simulink model "SplineGeneratorTest"  (R2016b)
settings: Solver=VariableStepAuto  StartTime=0.0  StopTime=10.0  RelTol=1e-3
settings Model: DataDictionary=DataDictionary.sldd  Creator=march  LastModifiedBy=Taeke

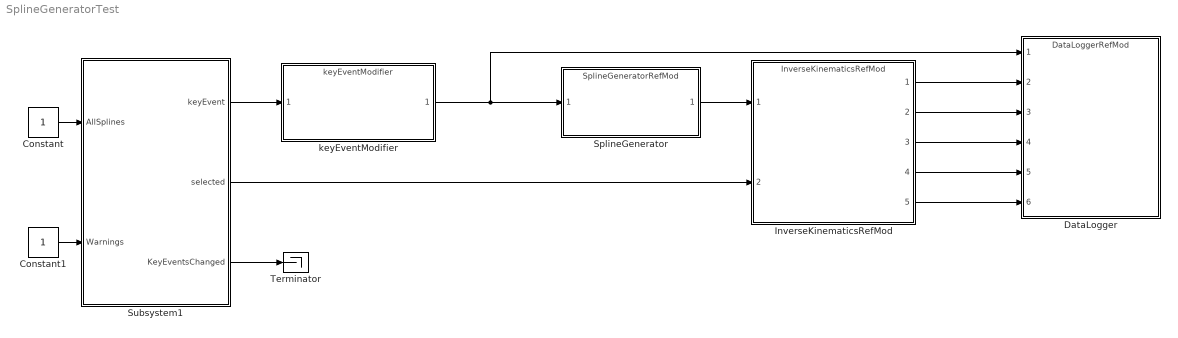
== system SplineGeneratorTest ==
  Constant : Constant
  Constant1 : Constant
  DataLogger : ModelReference  ModelNameDialog=DataLoggerRefMod.slx  SimulationMode=Normal  ModelReferenceVersion=1.16
  InverseKinematicsRefMod : ModelReference  ModelNameDialog=InverseKinematicsRefMod.slx  SimulationMode=Normal  ModelReferenceVersion=1.78
  SplineGenerator : ModelReference  ModelNameDialog=SplineGeneratorRefMod.slx  SimulationMode=Normal  ModelReferenceVersion=1.42
  Subsystem1 : Subsystem
  Terminator : Terminator
  keyEventModifier : ModelReference  ModelNameDialog=keyEventModifier.slx  SimulationMode=Normal  ModelReferenceVersion=1.7
  wires:
  Subsystem1/3(KeyEventsChanged) -> Terminator/1
  Constant/1 -> Subsystem1/1(AllSplines)
  Constant1/1 -> Subsystem1/2(Warnings)
  keyEventModifier/1 -> DataLogger/1, SplineGenerator/1
  SplineGenerator/1 -> InverseKinematicsRefMod/1
  Subsystem1/1(keyEvent) -> keyEventModifier/1
  Subsystem1/2(selected) -> InverseKinematicsRefMod/2
  InverseKinematicsRefMod/5 -> DataLogger/6
  InverseKinematicsRefMod/4 -> DataLogger/5
  InverseKinematicsRefMod/3 -> DataLogger/4
  InverseKinematicsRefMod/2 -> DataLogger/3
  InverseKinematicsRefMod/1 -> DataLogger/2

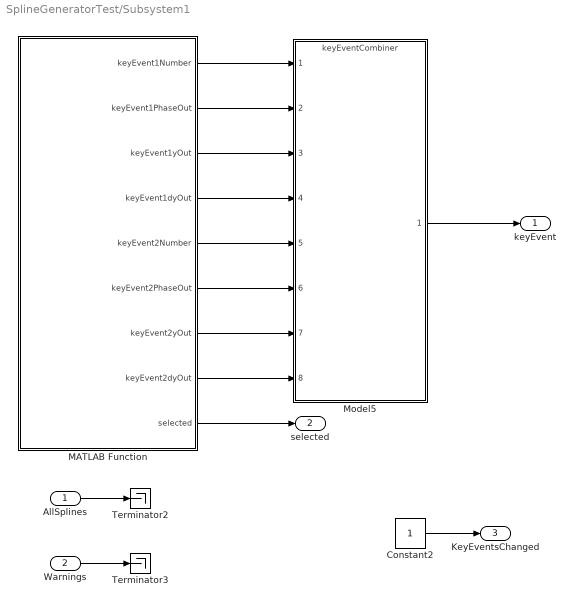
== system SplineGeneratorTest/Subsystem1 ==
  AllSplines : Inport
  Warnings : Inport  Port=2
  Constant2 : Constant
  MATLAB Function : MATLAB Function  TreatAsAtomicUnit=on
  Model5 : ModelReference  ModelNameDialog=keyEventCombiner.slx  SimulationMode=Normal  ModelReferenceVersion=1.6
  Terminator2 : Terminator
  Terminator3 : Terminator
  keyEvent : Outport
  selected : Outport  Port=2
  KeyEventsChanged : Outport  Port=3
  wires:
  Warnings/1 -> Terminator3/1
  MATLAB Function/8(keyEvent2dyOut) -> Model5/8
  AllSplines/1 -> Terminator2/1
  MATLAB Function/3(keyEvent1yOut) -> Model5/3
  Constant2/1 -> KeyEventsChanged/1
  MATLAB Function/4(keyEvent1dyOut) -> Model5/4
  MATLAB Function/2(keyEvent1PhaseOut) -> Model5/2
  MATLAB Function/6(keyEvent2PhaseOut) -> Model5/6
  MATLAB Function/1(keyEvent1Number) -> Model5/1
  MATLAB Function/7(keyEvent2yOut) -> Model5/7
  Model5/1 -> keyEvent/1
  MATLAB Function/5(keyEvent2Number) -> Model5/5
  MATLAB Function/9(selected) -> selected/1

== matlab function SplineGeneratorTest/Subsystem1/MATLAB Function ==
  data: keyEvent1Number output; keyEvent1PhaseOut output; keyEvent1yOut output; keyEvent1dyOut output; keyEvent2Number output; keyEvent2PhaseOut output; keyEvent2yOut output; keyEvent2dyOut output; selected output
function [keyEvent1Number, keyEvent1PhaseOut,keyEvent1yOut,keyEvent1dyOut, ...
    keyEvent2Number, keyEvent2PhaseOut,keyEvent2yOut,keyEvent2dyOut,...
    selected] = fcn()

selected1 = [0 ,1, 0, 0]; %[Hip, Knee, x, y];
selected2 = [0 ,0, 1, 0]; %[Hip, Knee, x, y];

selected = selected1 + selected2; %knee and x selected

keyEventHipPhase = [55, 85]; %hip angle: for test look_up_hip_y
keyEventHipAngle = [-7, 20]/180*pi; %hip angle: for test look_up_hip_y
keyEventHipdAngle = [0,0]; %hip angle: for test look_up_hip_y

keyEventKneePhase = [0, 18, 45, 78];   %knee angle: for test look_up_hip_y
keyEventKneeAngle = [0, 15, 2, 60]/180*pi;  %knee angle: for test look_up_hip_y 
keyEventKneedAngle = [0,0, 0 ,0]; %knee angle: for test look_up_hip_y

keyEventxPhase = [0, 18, 45, 62];
keyEventxPos = [0.15, 0.0, -0.1, -0.25]; %[m] x position: for test look_up_hip_y
keyEventxdPos = [0, -0.0035, -0.0035, 0]; % x position: for test look_up_hip_y

if selected1(1)
    keyEvent1Phase = keyEventHipPhase;
    keyEvent1y = keyEventHipAngle;
    keyEvent1dy = keyEventHipdAngle;
elseif selected1(2)
    keyEvent1Phase = keyEventKneePhase; 
    keyEvent1y = keyEventKneeAngle;
    keyEvent1dy = keyEventKneedAngle;
elseif selected1(3)  
    keyEvent1Phase = keyEventxPhase;
    keyEvent1y = keyEventxPos;
    keyEvent1dy = keyEventxdPos;
elseif selected1(4)    
    keyEvent1Phase = keyEventyPhase; 
    keyEvent1y = keyEventxPos;
    keyEvent1dy = keyEventxdAngle;
end

if selected2(1)
    keyEvent2Phase = keyEventHipPhase;
    keyEvent2y = keyEventHipAngle;
    keyEvent2dy = keyEventHipdAngle;
elseif selected2(2)
    keyEvent2Phase = keyEventKneePhase; 
    keyEvent2y = keyEventKneeAngle;
    keyEvent2dy = keyEventKneedAngle;
elseif selected2(3)  
    keyEvent2Phase = keyEventxPhase;
    keyEvent2y = keyEventxPos;
    keyEvent2dy = keyEventxdPos;
elseif selected2(4)    
    keyEvent2Phase = keyEventyPhase; 
    keyEvent2y = keyEventxPos;
    keyEvent2dy = keyEventxdAngle;
end

keyEvent1Number = length(keyEvent1Phase);
keyEvent1PhaseOut = [keyEvent1Phase, nan(1,20-keyEvent1Number)];
keyEvent1yOut = [keyEvent1y, nan(1,20-keyEvent1Number)];
keyEvent1dyOut = [keyEvent1dy, nan(1,20-keyEvent1Number)];

keyEvent2Number = length(keyEvent2Phase);
keyEvent2PhaseOut = [keyEvent2Phase, nan(1,20-keyEvent2Number)];
keyEvent2yOut = [keyEvent2y, nan(1,20-keyEvent2Number)];
keyEvent2dyOut = [keyEvent2dy, nan(1,20-keyEvent2Number)];

end
